simulink model "pi_control_sim"  (R2021b)
settings: Solver=ode4  StartTime=0.0  StopTime=10.0  FixedStep=0.001  RelTol=1e-3
values from neighbouring files (symbols this model uses):
  A = [ -R/L -K_hat/L 0 ... (first row only)    [dc_sim_inpgps.m]    (also in in_gps_est.m = [ -R_hat/L_hat -K/L_hat 0; untitled.m = [ -R_hat/L_hat -K_hat/L_hat 0)
  B = [ 1/L; 0 ; 0]    [dc_sim_inpgps.m]    (also in in_gps_est.m = [ 1/L_hat; 0 ; 0]; untitled.m = [ 1/L_hat; 0 ; 0])
  C = eye(3)    [dc_sim_inpgps.m]    (also in in_gps_est.m; untitled.m)
  D = [0;0;0;]    [dc_sim_inpgps.m]    (also in in_gps_est.m; untitled.m)
  K = K_hat(3)    [in_gps_est.m]    (also in untitled.m = 0.0603)
  Kac = 1/Kpc    [in_gps_est.m]
  Kas = 1/Kps    [in_gps_est.m]
  Kic = R_hat*wcc    [in_gps_est.m]
  Kis = J_hat*wcs^2/(5*K)    [in_gps_est.m]
  Kpc = L_hat*wcc    [in_gps_est.m]
  Kps = J_hat*wcs/K    [in_gps_est.m]
settings Model: Creator=JongBeom  LastModifiedBy=JongBeom
settings DataIOCC: ReturnWorkspaceOutputs=off

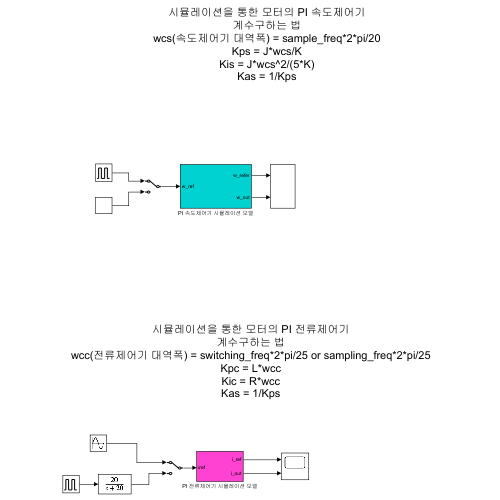
[thumbnail: Simulink's stored preview of the top-level diagram]
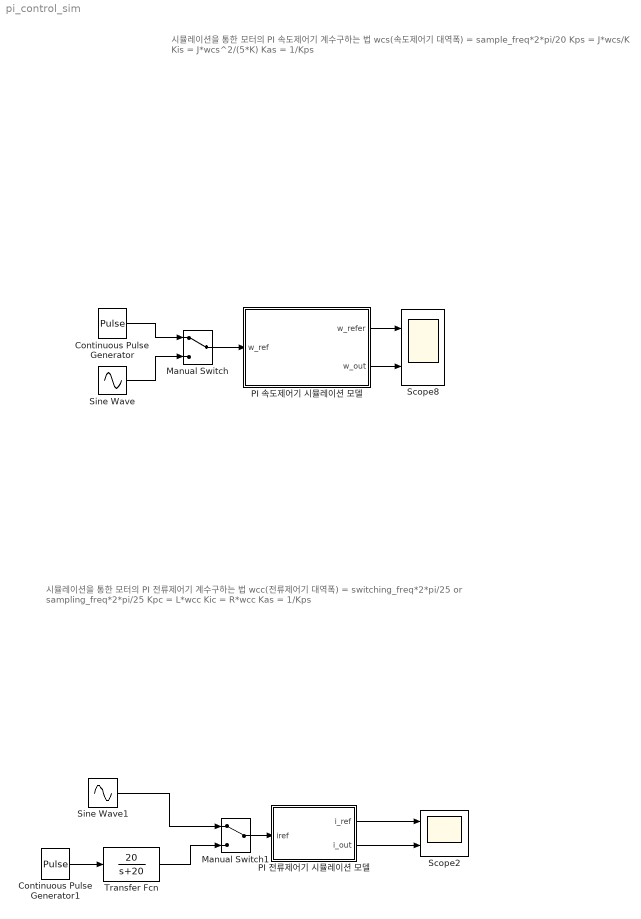
== system pi_control_sim ==
  note: 시뮬레이션을 통한 모터의 PI 전류제어기
      | 계수구하는 법
      | wcc(전류제어기 대역폭) = switching_freq*2*pi/25 or sampling_freq*2*pi/25
      | Kpc = L*wcc
      | Kic = R*wcc
      | Kas = 1/Kps
  note: 시뮬레이션을 통한 모터의 PI 속도제어기
      | 계수구하는 법
      | wcs(속도제어기 대역폭) = sample_freq*2*pi/20
      | Kps = J*wcs/K
      | Kis = J*wcs^2/(5*K)
      | Kas = 1/Kps
  Continuous Pulse Generator : DiscretePulseGenerator  PulseType=Time based  Amplitude=100  Period=10  PulseWidth=50
  Continuous Pulse Generator1 : DiscretePulseGenerator  PulseType=Time based  Amplitude=0.05  Period=10  PulseWidth=50
  Manual Switch : ManualSwitch
  Manual Switch1 : ManualSwitch
  PI 속도제어기 시뮬레이션 모델 : Subsystem
  PI 전류제어기 시뮬레이션 모델 : Subsystem
  Scope2 : Scope  NumInputPorts=2
  Scope8 : Scope  NumInputPorts=2
  Sine Wave : Sin  Amplitude=200  Frequency=5  SampleTime=0
  Sine Wave1 : Sin  Amplitude=0.05  Frequency=5  SampleTime=0
  Transfer Fcn : TransferFcn  Numerator=[20]  Denominator=[1 20]
  wires:
  Continuous Pulse Generator/1 -> Manual Switch/1
  Sine Wave/1 -> Manual Switch/2
  Manual Switch/1 -> PI 속도제어기 시뮬레이션 모델/1(w_ref)
  PI 속도제어기 시뮬레이션 모델/1(w_refer) -> Scope8/1
  PI 속도제어기 시뮬레이션 모델/2(w_out) -> Scope8/2
  Manual Switch1/1 -> PI 전류제어기 시뮬레이션 모델/1(iref)
  PI 전류제어기 시뮬레이션 모델/1(i_ref) -> Scope2/1
  PI 전류제어기 시뮬레이션 모델/2(i_out) -> Scope2/2
  Sine Wave1/1 -> Manual Switch1/1
  Transfer Fcn/1 -> Manual Switch1/2
  Continuous Pulse Generator1/1 -> Transfer Fcn/1

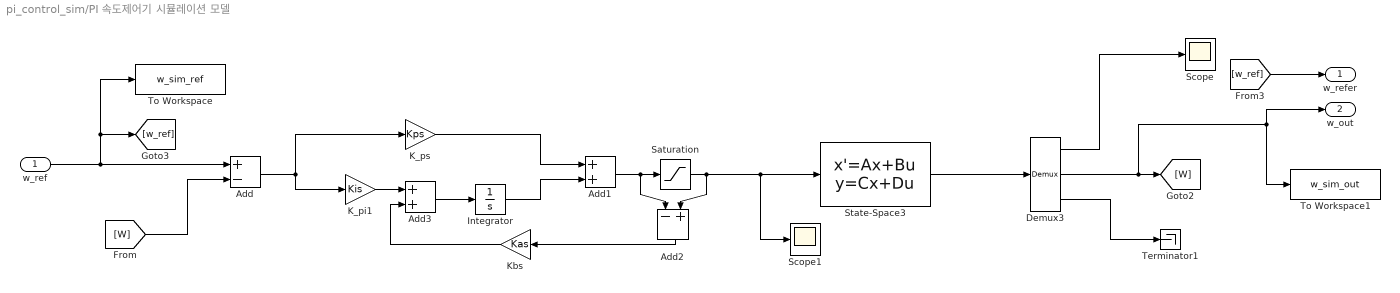
== system pi_control_sim/PI 속도제어기 시뮬레이션 모델 ==
  w_ref : Inport
  Add : Sum  Inputs=+-
  Add1 : Sum
  Add2 : Sum  Inputs=-+
  Add3 : Sum
  Demux3 : Demux  Outputs=3
  Integrator : Integrator
  K_pi1 : Gain  Gain=Kis
  K_ps : Gain  Gain=Kps
  Kbs : Gain  Gain=Kas
  Saturation : Saturate  UpperLimit=12  LowerLimit=-12
  Scope : Scope
  Scope1 : Scope
  State-Space3 : StateSpace  A=A  B=B  C=C  D=D  InitialCondition=0
  Terminator1 : Terminator
  To Workspace : ToWorkspace  VariableName=w_sim_ref  SampleTime=-1
  To Workspace1 : ToWorkspace  VariableName=w_sim_out  SampleTime=-1
  w_refer : Outport
  w_out : Outport  Port=2
  wires:
  Demux3/2 -> w_out/1, To Workspace1/1, [W]
  Demux3/3 -> Terminator1/1
  Saturation/1 -> Scope1/1, State-Space3/1, Add2/2
  Add2/1 -> Kbs/1
  Add3/1 -> Integrator/1
  w_ref/1 -> [w_ref], To Workspace/1, Add/1
  Demux3/1 -> Scope/1
  [W] -> Add/2
  Add1/1 -> Add2/1, Saturation/1
  K_pi1/1 -> Add3/1
  Kbs/1 -> Add3/2
  K_ps/1 -> Add1/1
  Integrator/1 -> Add1/2
  Add/1 -> K_ps/1, K_pi1/1
  State-Space3/1 -> Demux3/1
  [w_ref] -> w_refer/1

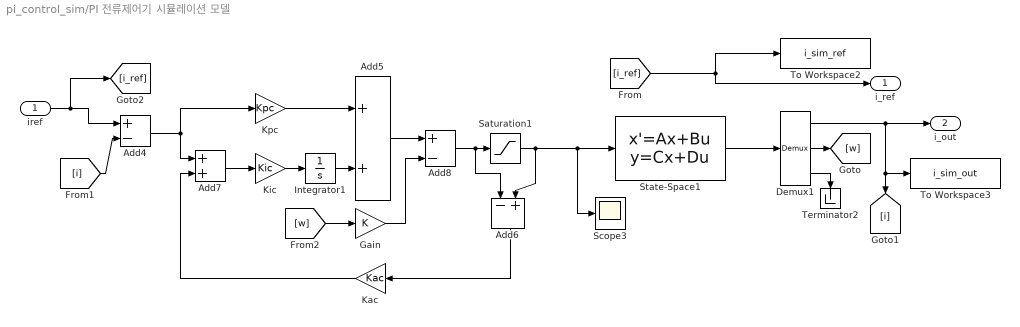
== system pi_control_sim/PI 전류제어기 시뮬레이션 모델 ==
  iref : Inport
  Add4 : Sum  Inputs=+-
  Add5 : Sum
  Add6 : Sum  Inputs=-+
  Add7 : Sum
  Add8 : Sum  Inputs=+-
  Demux1 : Demux  Outputs=3
  Gain : Gain  Gain=K
  Integrator1 : Integrator
  Kac : Gain  Gain=Kac
  Kic : Gain  Gain=Kic
  Kpc : Gain  Gain=Kpc
  Saturation1 : Saturate  UpperLimit=12  LowerLimit=-12
  Scope3 : Scope
  State-Space1 : StateSpace  A=A  B=B  C=C  D=D  InitialCondition=0
  Terminator2 : Terminator
  To Workspace2 : ToWorkspace  VariableName=i_sim_ref  SampleTime=-1
  To Workspace3 : ToWorkspace  VariableName=i_sim_out  SampleTime=-1
  i_ref : Outport
  i_out : Outport  Port=2
  wires:
  Add8/1 -> Saturation1/1, Add6/1
  State-Space1/1 -> Demux1/1
  [i] -> Add4/2
  Demux1/1 -> To Workspace3/1, [i], i_out/1
  Add6/1 -> Kac/1
  [i_ref] -> i_ref/1, To Workspace2/1
  Integrator1/1 -> Add5/2
  Kpc/1 -> Add5/1
  Kic/1 -> Integrator1/1
  Gain/1 -> Add8/2
  Saturation1/1 -> Scope3/1, State-Space1/1, Add6/2
  Kac/1 -> Add7/2
  Add4/1 -> Add7/1, Kpc/1
  Add7/1 -> Kic/1
  Demux1/3 -> Terminator2/1
  Add5/1 -> Add8/1
  Demux1/2 -> [w]
  iref/1 -> [i_ref], Add4/1
  [w] -> Gain/1
